simulink model "Proj2_P1"  (Simulink 8.6)
settings: Solver=ode45  StartTime=0.0  StopTime=25  MaxStep=0.001  RelTol=1e-3
values from neighbouring files (symbols this model uses):
  fl_rd_0 = fl_rd_rated    [Proj2_IM_IC_rated.m]    (also in Proj2_P1_calc.m = eps)
  fl_sd_0 = fl_sd_rated    [Proj2_IM_IC_rated.m]    (also in Proj2_P1_calc.m = 0)
  fl_sq_0 = fl_sq_rated    [Proj2_IM_IC_rated.m]    (also in Proj2_P1_calc.m = 0)
  Ia_0 = 0    [Proj2_P1_calc.m]
  IA_0 = 0    [Proj2_P1_calc.m]
  Ib_0 = 0    [Proj2_P1_calc.m]
  IB_0 = 0    [Proj2_P1_calc.m]
  Ic_0 = 0    [Proj2_P1_calc.m]
  IC_0 = 0    [Proj2_P1_calc.m]
  J_eq = 75    [Proj2_IM_parameters.m]
  L_lr = X_lr/w_syn    (= 8.22300539308e-05)    [Proj2_IM_parameters.m]
  L_ls = X_ls/w_syn    (= 9.01878010854e-05)    [Proj2_IM_parameters.m]
  L_m = X_m /w_syn    (= 0.00152788745368)    [Proj2_IM_parameters.m]
  L_r = L_lr+L_m    (= 0.00161011750761)    [Proj2_IM_parameters.m]
  L_s = L_ls+L_m    (= 0.00161807525477)    [Proj2_IM_parameters.m]
  p = 6    [Proj2_IM_parameters.m]
  R_r = 0.991*10^-3    (= 0.000991)    [Proj2_IM_parameters.m]
  R_s = 1.4*10^-3    (= 0.0014)    [Proj2_IM_parameters.m]
  T_L_0 = T_L_rated    [Proj2_IM_IC_rated.m]    (also in Proj2_P1_calc.m = 0)
  T_L_rated = T_em_rated    [Proj2_IM_parameters.m]
  tau_r = L_r/R_r    (= 1.62474016914)    [Proj2_IM_parameters.m]
  theta_Aa_0 = 0    [Proj2_P1_calc.m]
  theta_da_0 = theta_fl_rated_a    [Proj2_IM_IC_rated.m]    (also in Proj2_P1_calc.m = 0)
  theta_dA_0 = theta_fl_rated_a    [Proj2_IM_IC_rated.m]    (also in Proj2_P1_calc.m = 0)
  V_ll_rated = 575    [Proj2_IM_parameters.m]
  Va_0 = 0    [Proj2_P1_calc.m]
  Vb_0 = 0    [Proj2_P1_calc.m]
  Vc_0 = 0    [Proj2_P1_calc.m]
  w_mech_0 = w_mech_rated    [Proj2_IM_IC_rated.m]    (also in Proj2_P1_calc.m = 0)
libraries: aerolibutil x8
settings Model: Creator=XP  LastModifiedBy=XP
settings DataIOCC: SaveFormat=Dataset  SignalLoggingSaveFormat=Dataset
settings OptimizationCC: ExpressionDepthLimit=128
settings DebuggingCC: UnderspecifiedInitializationDetection=Simplified  MergeDetectMultiDrivingBlocksExec=error  SolverPrmCheckMsg=none  FcnCallInpInsideContextMsg=EnableAllAsError  StateNameClashWarn=none
settings HardwareCC: ProdBitPerPointer=64  ProdLargestAtomicFloat=Float  ProdIntDivRoundTo=Zero  ProdEndianess=LittleEndian  ProdWordSize=64  ProdHWDeviceType=Intel->x86-64 (Windows64)
settings GRTTargetCC: GeneratePreprocessorConditionals=Use local settings  CombineOutputUpdateFcns=on  GRTInterface=off
settings ConfigComp: CovModelRefEnable=off

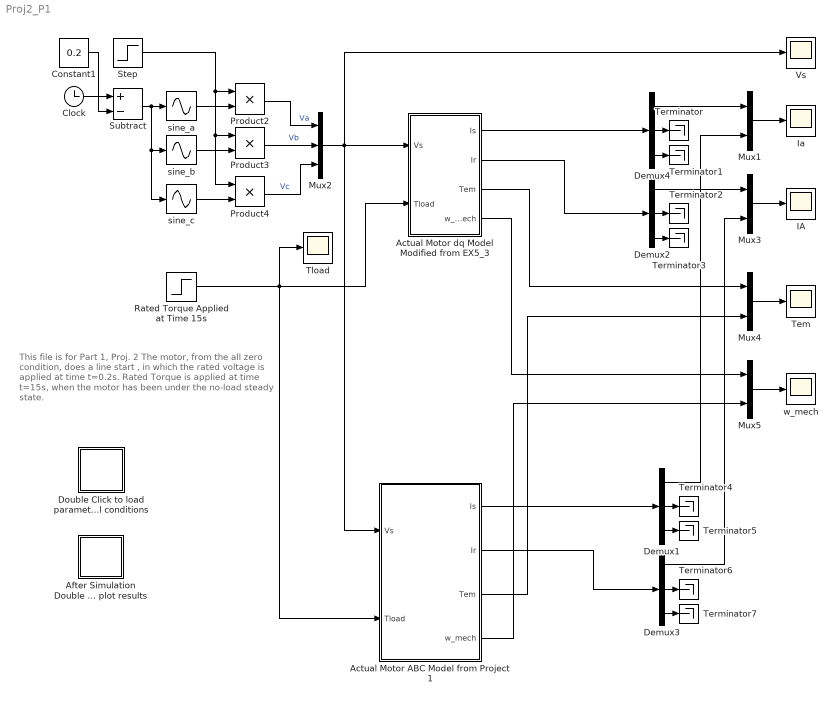
== system Proj2_P1 ==
  note: This file is for Part 1, Proj. 2
      |
      | The motor, from the all zero condition, does a line start ,
      | in which the rated voltage is applied at time t=0.2s.
      |
      | Rated Torque is applied at time t=15s,
      | when the motor has been under the no-load steady state.
  "Actual Motor ABC Model from Project 1 " : Subsystem
  Actual Motor dq Model Modified from EX5_3 : Subsystem
  After Simulation Double Click to plot results : Subsystem
      settings: OpenFcn=Proj2_P1_plots
      mask Display:
      | plot(0,0)
      | plot(100,100)
      | disp('Plot')
  Clock : Clock
  Constant1 : Constant  Value=0.2
  Demux{1..4} (4 alike) : Demux  Outputs=3
  Double Click to load parameters and initial conditions : Subsystem
      settings: OpenFcn=Proj2_P1_calc
      mask Display:
      | plot(0,0)
      | plot(100,100)
      | disp('Start')
  IA : Scope
  Ia : Scope
  Mux{1,3..5} (4 alike) : Mux  Inputs=2
  Mux2 : Mux  Inputs=3
  Product2 : Product
  Product3 : Product
  Product4 : Product
  Rated Torque Applied at Time 15s : Step  Time=15  Before=T_L_0  After=T_L_rated  SampleTime=0
  Step : Step  Time=0.2  SampleTime=0
  Subtract : Sum  Inputs=+-
  Tem : Scope
  Terminator{,1..7} (8 alike) : Terminator
  Tload : Scope
  Vs : Scope
  sine_a : Sin  TimeSource=Use external signal  Amplitude=V_ll_rated*sqrt(2/3)  Frequency=60*2*pi  Phase=pi/2  SampleTime=0
  sine_b : Sin  TimeSource=Use external signal  Amplitude=V_ll_rated*sqrt(2/3)  Frequency=60*2*pi  Phase=pi/2-2*pi/3  SampleTime=0
  sine_c : Sin  TimeSource=Use external signal  Amplitude=V_ll_rated*sqrt(2/3)  Frequency=60*2*pi  Phase=pi/2-4*pi/3  SampleTime=0
  w_mech : Scope
  wires:
  Subtract/1 -> sine_c/1, sine_b/1, sine_a/1
  Step/1 -> Product3/1, Product4/1, Product2/1
  sine_a/1 -> Product2/2
  Product2/1 -> Mux2/1  "Va"
  sine_c/1 -> Product4/2
  sine_b/1 -> Product3/2
  Product3/1 -> Mux2/2  "Vb"
  Product4/1 -> Mux2/3  "Vc"
  Clock/1 -> Subtract/1
  Constant1/1 -> Subtract/2
  Mux2/1 -> "Actual Motor ABC Model from Project 1 "/1(Vs), Actual Motor dq Model Modified from EX5_3/1(Vs), Vs/1
  Rated Torque Applied at Time 15s/1 -> Tload/1, Actual Motor dq Model Modified from EX5_3/2(Tload), "Actual Motor ABC Model from Project 1 "/2(Tload)
  Actual Motor dq Model Modified from EX5_3/1(Is) -> Demux4/1
  "Actual Motor ABC Model from Project 1 "/1(Is) -> Demux1/1
  Actual Motor dq Model Modified from EX5_3/2(Ir) -> Demux2/1
  "Actual Motor ABC Model from Project 1 "/2(Ir) -> Demux3/1
  Demux4/1 -> Mux1/1
  Demux1/1 -> Mux1/2
  Mux1/1 -> Ia/1
  Actual Motor dq Model Modified from EX5_3/3(Tem) -> Mux4/1
  "Actual Motor ABC Model from Project 1 "/3(Tem) -> Mux4/2
  Mux4/1 -> Tem/1
  Mux5/1 -> w_mech/1
  Actual Motor dq Model Modified from EX5_3/4(w_mech) -> Mux5/1
  "Actual Motor ABC Model from Project 1 "/4(w_mech) -> Mux5/2
  Mux3/1 -> IA/1
  Demux2/1 -> Mux3/1
  Demux3/1 -> Mux3/2
  Demux4/2 -> Terminator/1
  Demux4/3 -> Terminator1/1
  Demux2/2 -> Terminator2/1
  Demux2/3 -> Terminator3/1
  Demux1/2 -> Terminator4/1
  Demux1/3 -> Terminator5/1
  Demux3/2 -> Terminator6/1
  Demux3/3 -> Terminator7/1

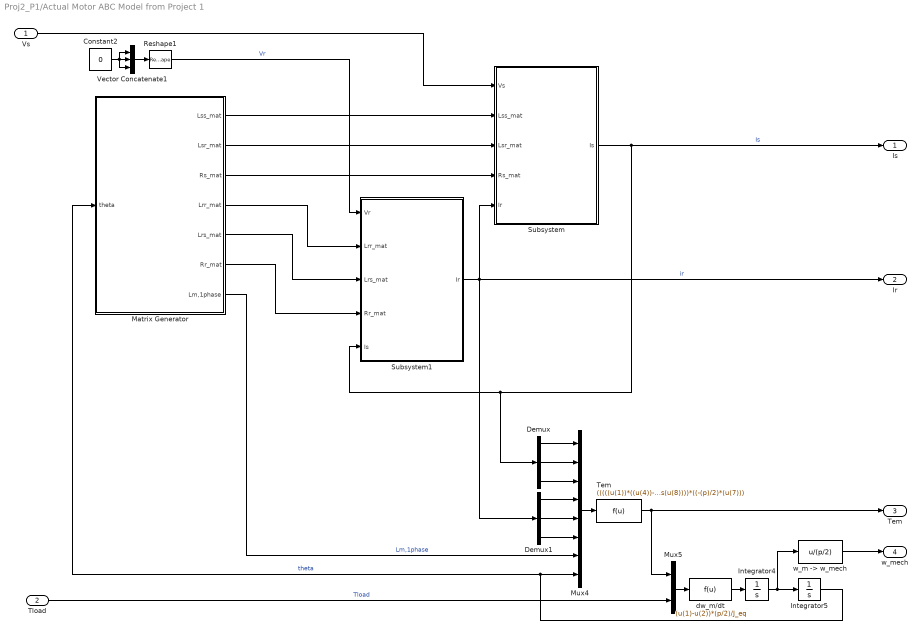
== system Proj2_P1/Actual Motor ABC Model from Project 1  ==
  Vs : Inport
  Tload : Inport  Port=2
  Constant2 : Constant  Value=0
  Demux : Demux  Outputs=3
  Demux1 : Demux  Outputs=3
  Integrator4 : Integrator  InitialCondition=w_mech_0*p/2
  Integrator5 : Integrator  InitialCondition=theta_Aa_0
  Matrix Generator : Subsystem
  Mux4 : Mux  Inputs=8
  Mux5 : Mux  Inputs=2
  Reshape1 : Reshape  OutputDimensionality=Customize  OutputDimensions=[3,1]
  Subsystem : Subsystem
  Subsystem1 : Subsystem
  "Tem " : Fcn  Expr=(((((u(1))*((u(4))-(0.5*(u(5)))-(0.5*(u(6)))))+((u(2))*((u(5))-(0.5*(u(4)))-(0.5*(u(6)))))+((u(3))*((u(6))-(0.5*(u(5)))-(0.5*(u(4))))))*sin(u(8)))+((sqrt(3)/2)*(((u(1))*((u(5))-(u(6))))+((u(2))*((u(6))-(u(4))))+((u(3))*((u(4))-(u(5)))))*cos(u(8))))*((-(p)/2)*(u(7)))
  Vector Concatenate1 : Concatenate  NumInputs=3
  dw_m/dt : Fcn  Expr=(u(1)-u(2))*(p/2)/J_eq
  "w_m -> w_mech" : Fcn  Expr=u/(p/2)
  Is : Outport
  Ir : Outport  Port=2
  Tem : Outport  Port=3
  w_mech : Outport  Port=4
  wires:
  Matrix Generator/7(Lm,1phase) -> Mux4/7  "Lm,1phase"
  Tload/1 -> Mux5/2  "Tload"
  Subsystem1/1(Ir) -> Ir/1, Demux1/1, Subsystem/5(Ir)  "ir"
  Integrator5/1 -> Mux4/8, Matrix Generator/1(theta)  "theta"
  Vector Concatenate1/1 -> Reshape1/1
  Reshape1/1 -> Subsystem1/1(Vr)  "Vr"
  Matrix Generator/5(Lrs_mat) -> Subsystem1/3(Lrs_mat)
  "w_m -> w_mech"/1 -> w_mech/1
  Demux/3 -> Mux4/3
  Demux1/1 -> Mux4/4
  Mux5/1 -> dw_m/dt/1
  Constant2/1 -> Vector Concatenate1/3, Vector Concatenate1/1, Vector Concatenate1/2
  Subsystem/1(Is) -> Is/1, Demux/1, Subsystem1/5(Is)  "Is"
  Matrix Generator/6(Rr_mat) -> Subsystem1/4(Rr_mat)
  Matrix Generator/4(Lrr_mat) -> Subsystem1/2(Lrr_mat)
  Demux1/2 -> Mux4/5
  Demux1/3 -> Mux4/6
  Mux4/1 -> "Tem "/1
  "Tem "/1 -> Tem/1, Mux5/1
  Demux/1 -> Mux4/1
  Demux/2 -> Mux4/2
  Integrator4/1 -> "w_m -> w_mech"/1, Integrator5/1
  dw_m/dt/1 -> Integrator4/1
  Matrix Generator/1(Lss_mat) -> Subsystem/2(Lss_mat)
  Matrix Generator/3(Rs_mat) -> Subsystem/4(Rs_mat)
  Matrix Generator/2(Lsr_mat) -> Subsystem/3(Lsr_mat)
  Vs/1 -> Subsystem/1(Vs)

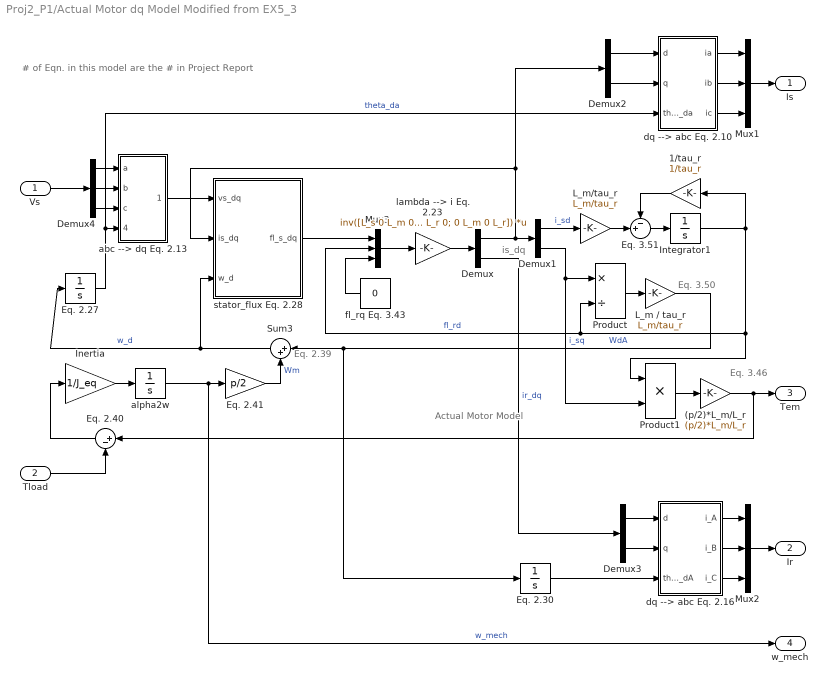
== system Proj2_P1/Actual Motor dq Model Modified from EX5_3 ==
  note: Eq. 2.39
  note: Eq. 3.46
  note: Eq. 3.50
  note: # of Eqn. in this model are the # in Project Report
  note: Actual Motor Model
  note: is_dq
  Vs : Inport
  Tload : Inport  Port=2
  (p/2)*L_m/L_r : Gain  Gain=(p/2)*L_m/L_r  SaturateOnIntegerOverflow=on  OutDataTypeStr=Inherit: Same as input  ParamDataTypeStr=Inherit: Same as input
  1/tau_r : Gain  Gain=1/tau_r  SaturateOnIntegerOverflow=on  OutDataTypeStr=Inherit: Same as input  ParamDataTypeStr=Inherit: Same as input
  Demux{,1..3} (4 alike) : Demux  Outputs=2
  Demux4 : Demux  Outputs=3
  Eq. 2.27 : Integrator  InitialCondition=theta_da_0
  Eq. 2.30 : Integrator  InitialCondition=theta_dA_0
  Eq. 2.40 : Sum  Inputs=|+-  SaturateOnIntegerOverflow=on  InputSameDT=on  OutDataTypeStr=Inherit: Same as first input
  Eq. 2.41 : Gain  Gain=p/2  SaturateOnIntegerOverflow=on  OutDataTypeStr=Inherit: Same as input  ParamDataTypeStr=Inherit: Same as input
  Eq. 3.51 : Sum  Inputs=-+|  SaturateOnIntegerOverflow=on  InputSameDT=on  OutDataTypeStr=Inherit: Same as first input
  Inertia : Gain  Gain=1/J_eq  SaturateOnIntegerOverflow=on  OutDataTypeStr=Inherit: Same as input  ParamDataTypeStr=Inherit: Same as input
  Integrator1 : Integrator  InitialCondition=fl_rd_0
  L_m / tau_r : Gain  Gain=L_m/tau_r  SaturateOnIntegerOverflow=on  OutDataTypeStr=Inherit: Same as input  ParamDataTypeStr=Inherit: Same as input
  L_m/tau_r : Gain  Gain=L_m/tau_r  SaturateOnIntegerOverflow=on  OutDataTypeStr=Inherit: Same as input  ParamDataTypeStr=Inherit: Same as input
  Mux1 : Mux  Inputs=3
  Mux2 : Mux  Inputs=3
  Mux3 : Mux  Inputs=3
  Product : Product  Inputs=*/  SaturateOnIntegerOverflow=on  RndMeth=Zero  InputSameDT=on  OutDataTypeStr=Inherit: Same as first input
  Product1 : Product  SaturateOnIntegerOverflow=on  RndMeth=Zero  InputSameDT=on  OutDataTypeStr=Inherit: Same as first input
  Sum3 : Sum  Inputs=|++  SaturateOnIntegerOverflow=on  InputSameDT=on  OutDataTypeStr=Inherit: Same as first input
  abc --> dq Eq. 2.13 : Subsystem
  alpha2w : Integrator  InitialCondition=w_mech_0
  dq --> abc Eq. 2.10 : Subsystem
  "dq --> abc Eq. 2.16 " : Subsystem
  fl_rq Eq. 3.43 : Constant  Value=0
  lambda --> i Eq. 2.23 : Gain  Gain=inv([L_s 0 L_m 0; 0 L_s 0 L_m; L_m 0 L_r 0; 0 L_m 0 L_r])  Multiplication=Matrix(K*u)  SaturateOnIntegerOverflow=on  OutDataTypeStr=Inherit: Same as input  ParamDataTypeStr=Inherit: Same as input
  stator_flux Eq. 2.28 : Subsystem
  Is : Outport
  Ir : Outport  Port=2
  Tem : Outport  Port=3
  w_mech : Outport  Port=4
  wires:
  Mux3/1 -> lambda --> i Eq. 2.23/1
  Demux/1 -> Demux1/1, stator_flux Eq. 2.28/2(is_dq), Demux2/1
  Eq. 2.27/1 -> dq --> abc Eq. 2.10/3(theta_da), abc --> dq Eq. 2.13/4(theta_da)  "theta_da"
  stator_flux Eq. 2.28/1(fl_s_dq) -> Mux3/1
  abc --> dq Eq. 2.13/1(vs_dq) -> stator_flux Eq. 2.28/1(vs_dq)
  lambda --> i Eq. 2.23/1 -> Demux/1
  Demux1/1 -> L_m/tau_r/1  "i_sd"
  L_m/tau_r/1 -> Eq. 3.51/2
  1/tau_r/1 -> Eq. 3.51/1
  Eq. 3.51/1 -> Integrator1/1
  Demux1/2 -> Product/1, Product1/2  "i_sq"
  Product/1 -> L_m / tau_r/1
  L_m / tau_r/1 -> Sum3/1, Eq. 2.30/1  "WdA"
  Product1/1 -> (p/2)*L_m/L_r/1
  fl_rq Eq. 3.43/1 -> Mux3/3
  Sum3/1 -> Eq. 2.27/1, stator_flux Eq. 2.28/3(w_d)  "w_d"
  (p/2)*L_m/L_r/1 -> Tem/1, Eq. 2.40/1
  Demux2/1 -> dq --> abc Eq. 2.10/1(d)
  Demux2/2 -> dq --> abc Eq. 2.10/2(q)
  dq --> abc Eq. 2.10/1(ia) -> Mux1/1
  dq --> abc Eq. 2.10/2(ib) -> Mux1/2
  dq --> abc Eq. 2.10/3(ic) -> Mux1/3
  Integrator1/1 -> 1/tau_r/1, Mux3/2, Product/2, Product1/1  "fl_rd"
  Eq. 2.41/1 -> Sum3/2  "Wm"
  Demux/2 -> Demux3/1  "ir_dq"
  Eq. 2.40/1 -> Inertia/1
  Inertia/1 -> alpha2w/1
  alpha2w/1 -> w_mech/1, Eq. 2.41/1  "w_mech"
  Tload/1 -> Eq. 2.40/2
  Mux1/1 -> Is/1
  Demux3/1 -> "dq --> abc Eq. 2.16 "/1(d)
  Demux3/2 -> "dq --> abc Eq. 2.16 "/2(q)
  Eq. 2.30/1 -> "dq --> abc Eq. 2.16 "/3(theta_dA)
  "dq --> abc Eq. 2.16 "/1(i_A) -> Mux2/1
  "dq --> abc Eq. 2.16 "/2(i_B) -> Mux2/2
  "dq --> abc Eq. 2.16 "/3(i_C) -> Mux2/3
  Mux2/1 -> Ir/1
  Demux4/1 -> abc --> dq Eq. 2.13/1(a)
  Demux4/2 -> abc --> dq Eq. 2.13/2(b)
  Demux4/3 -> abc --> dq Eq. 2.13/3(c)
  Vs/1 -> Demux4/1

== system Proj2_P1/After Simulation Double Click to plot results ==

== system Proj2_P1/Double Click to load parameters and initial conditions ==

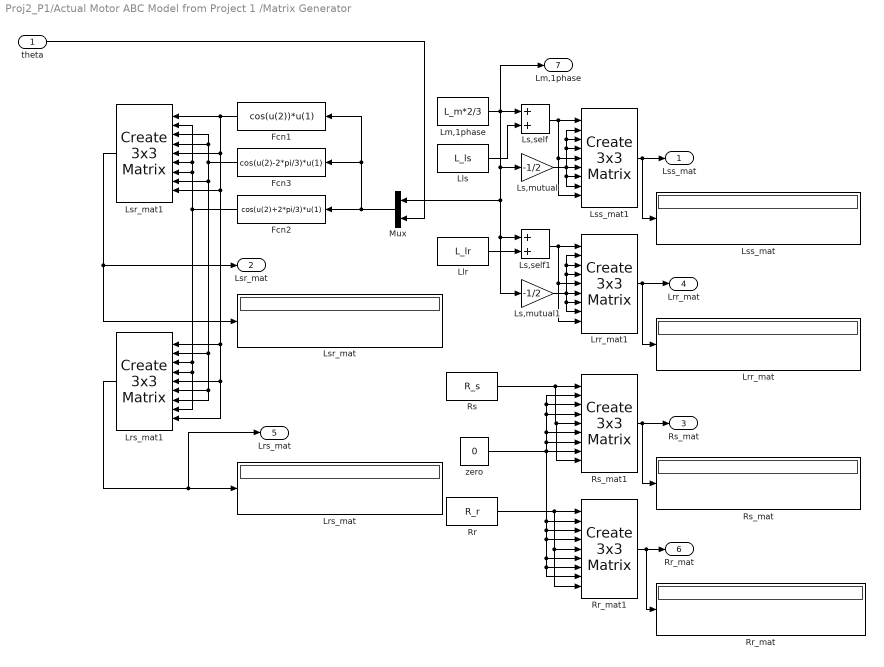
== system Proj2_P1/Actual Motor ABC Model from Project 1 /Matrix Generator ==
  theta : Inport
  Fcn1 : Fcn  Expr=cos(u(2))*u(1)
  Fcn2 : Fcn  Expr=cos(u(2)+2*pi/3)*u(1)
  Fcn3 : Fcn  Expr=cos(u(2)-2*pi/3)*u(1)
  Llr : Constant  Value=L_lr
  Lls : Constant  Value=L_ls
  "Lm,1phase " : Constant  Value=L_m*2/3
  "Lrr_mat " : Display
  Lrr_mat1 : aerolibutil/Create 3x3 Matrix
  "Lrs_mat " : Display
  Lrs_mat1 : aerolibutil/Create 3x3 Matrix
  Ls,mutual : Gain  Gain=-1/2
  Ls,mutual1 : Gain  Gain=-1/2
  Ls,self : Sum
  Ls,self1 : Sum
  "Lsr_mat " : Display
  Lsr_mat1 : aerolibutil/Create 3x3 Matrix
  "Lss_mat " : Display
  Lss_mat1 : aerolibutil/Create 3x3 Matrix
  Mux : Mux  Inputs=2
  "Rr " : Constant  Value=R_r
  "Rr_mat " : Display
  Rr_mat1 : aerolibutil/Create 3x3 Matrix
  Rs : Constant  Value=R_s
  "Rs_mat " : Display
  Rs_mat1 : aerolibutil/Create 3x3 Matrix
  "zero " : Constant  Value=0
  Lss_mat : Outport
  Lsr_mat : Outport  Port=2
  Rs_mat : Outport  Port=3
  Lrr_mat : Outport  Port=4
  Lrs_mat : Outport  Port=5
  Rr_mat : Outport  Port=6
  Lm,1phase : Outport  Port=7
  wires:
  Ls,self/1 -> Lss_mat1/1, Lss_mat1/9, Lss_mat1/5
  Lls/1 -> Ls,self/2
  Lsr_mat1/1 -> Lsr_mat/1, "Lsr_mat "/1
  Mux/1 -> Fcn3/1, Fcn1/1, Fcn2/1
  Rs/1 -> Rs_mat1/9, Rs_mat1/5, Rs_mat1/1
  "Rr "/1 -> Rr_mat1/9, Rr_mat1/5, Rr_mat1/1
  Lrs_mat1/1 -> Lrs_mat/1, "Lrs_mat "/1
  Fcn1/1 -> Lrs_mat1/1, Lrs_mat1/5, Lrs_mat1/9, Lsr_mat1/9, Lsr_mat1/5, Lsr_mat1/1
  Lrr_mat1/1 -> Lrr_mat/1, "Lrr_mat "/1
  Ls,mutual/1 -> Lss_mat1/8, Lss_mat1/7, Lss_mat1/4, Lss_mat1/3, Lss_mat1/2, Lss_mat1/6
  Rr_mat1/1 -> Rr_mat/1, "Rr_mat "/1
  Ls,self1/1 -> Lrr_mat1/9, Lrr_mat1/5, Lrr_mat1/1
  "zero "/1 -> Rs_mat1/4, Rs_mat1/3, Rs_mat1/2, Rs_mat1/6, Rs_mat1/7, Rr_mat1/2, Rr_mat1/3, Rr_mat1/4, Rr_mat1/6, Rr_mat1/7, Rr_mat1/8, Rs_mat1/8
  Fcn3/1 -> Lrs_mat1/7, Lrs_mat1/6, Lrs_mat1/2, Lsr_mat1/8, Lsr_mat1/4, Lsr_mat1/3
  Llr/1 -> Ls,self1/2
  Rs_mat1/1 -> Rs_mat/1, "Rs_mat "/1
  Ls,mutual1/1 -> Lrr_mat1/8, Lrr_mat1/7, Lrr_mat1/4, Lrr_mat1/3, Lrr_mat1/2, Lrr_mat1/6
  Fcn2/1 -> Lsr_mat1/7, Lsr_mat1/6, Lsr_mat1/2, Lrs_mat1/8, Lrs_mat1/4, Lrs_mat1/3
  theta/1 -> Mux/2
  "Lm,1phase "/1 -> Lm,1phase/1, Mux/1, Ls,self1/1, Ls,mutual1/1, Ls,mutual/1, Ls,self/1
  Lss_mat1/1 -> Lss_mat/1, "Lss_mat "/1

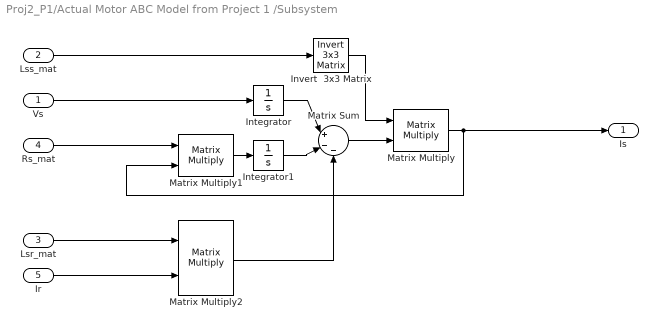
== system Proj2_P1/Actual Motor ABC Model from Project 1 /Subsystem ==
  Vs : Inport
  Lss_mat : Inport  Port=2
  Lsr_mat : Inport  Port=3
  Rs_mat : Inport  Port=4
  Ir : Inport  Port=5
  Integrator : Integrator  InitialCondition=[Va_0;Vb_0;Vc_0]
  Integrator1 : Integrator  InitialCondition=R_s*eye(3)*[Ia_0;Ib_0;Ic_0]
  Invert  3x3 Matrix : aerolibutil/Invert  3x3 Matrix
  Matrix Sum : Sum  Inputs=|+--
  Matrix Multiply : Product  Multiplication=Matrix(*)
  Matrix Multiply1 : Product  Multiplication=Matrix(*)
  Matrix Multiply2 : Product  Multiplication=Matrix(*)
  Is : Outport
  wires:
  Matrix Sum/1 -> Matrix Multiply/2
  Matrix Multiply/1 -> Is/1, Matrix Multiply1/2
  Matrix Multiply2/1 -> Matrix Sum/3
  Lss_mat/1 -> Invert  3x3 Matrix/1
  Vs/1 -> Integrator/1
  Invert  3x3 Matrix/1 -> Matrix Multiply/1
  Integrator/1 -> Matrix Sum/1
  Lsr_mat/1 -> Matrix Multiply2/1
  Matrix Multiply1/1 -> Integrator1/1
  Integrator1/1 -> Matrix Sum/2
  Rs_mat/1 -> Matrix Multiply1/1
  Ir/1 -> Matrix Multiply2/2

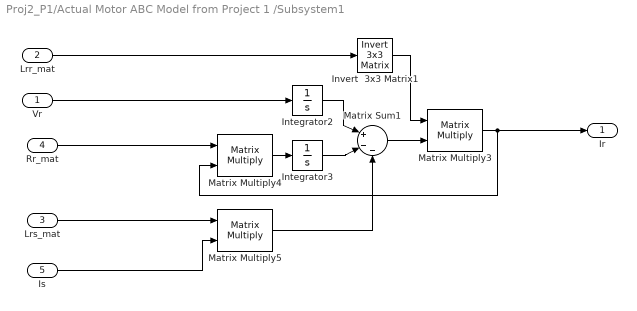
== system Proj2_P1/Actual Motor ABC Model from Project 1 /Subsystem1 ==
  Vr : Inport
  Lrr_mat : Inport  Port=2
  Lrs_mat : Inport  Port=3
  Rr_mat : Inport  Port=4
  Is : Inport  Port=5
  Integrator2 : Integrator
  Integrator3 : Integrator  InitialCondition=R_r*eye(3)*[IA_0;IB_0;IC_0]
  Invert  3x3 Matrix1 : aerolibutil/Invert  3x3 Matrix
  Matrix Sum1 : Sum  Inputs=|+--
  Matrix Multiply3 : Product  Multiplication=Matrix(*)
  Matrix Multiply4 : Product  Multiplication=Matrix(*)
  Matrix Multiply5 : Product  Multiplication=Matrix(*)
  Ir : Outport
  wires:
  Integrator3/1 -> Matrix Sum1/2
  Rr_mat/1 -> Matrix Multiply4/1
  Matrix Multiply4/1 -> Integrator3/1
  Is/1 -> Matrix Multiply5/2
  Invert  3x3 Matrix1/1 -> Matrix Multiply3/1
  Matrix Sum1/1 -> Matrix Multiply3/2
  Matrix Multiply3/1 -> Ir/1, Matrix Multiply4/2
  Integrator2/1 -> Matrix Sum1/1
  Vr/1 -> Integrator2/1
  Lrr_mat/1 -> Invert  3x3 Matrix1/1
  Lrs_mat/1 -> Matrix Multiply5/1
  Matrix Multiply5/1 -> Matrix Sum1/3

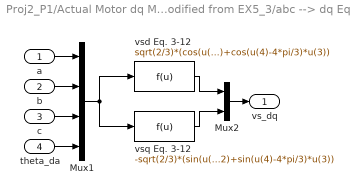
== system Proj2_P1/Actual Motor dq Model Modified from EX5_3/abc --> dq Eq. 2.13 ==
  a : Inport
  b : Inport  Port=2
  c : Inport  Port=3
  theta_da : Inport  Port=4
  Mux1 : Mux
  Mux2 : Mux  Inputs=2
  vsd Eq. 3-12 : Fcn  Expr=sqrt(2/3)*(cos(u(4))*u(1)+cos(u(4)-2*pi/3)*u(2)+cos(u(4)-4*pi/3)*u(3))
  vsq Eq. 3-12 : Fcn  Expr=-sqrt(2/3)*(sin(u(4))*u(1)+sin(u(4)-2*pi/3)*u(2)+sin(u(4)-4*pi/3)*u(3))
  vs_dq : Outport
  wires:
  Mux1/1 -> vsd Eq. 3-12/1, vsq Eq. 3-12/1
  vsd Eq. 3-12/1 -> Mux2/1
  vsq Eq. 3-12/1 -> Mux2/2
  a/1 -> Mux1/1
  b/1 -> Mux1/2
  c/1 -> Mux1/3
  theta_da/1 -> Mux1/4
  Mux2/1 -> vs_dq/1

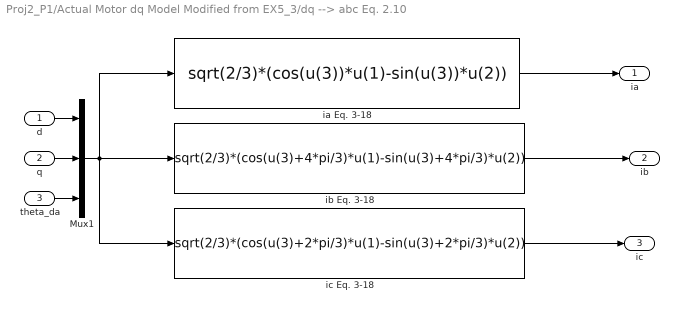
== system Proj2_P1/Actual Motor dq Model Modified from EX5_3/dq --> abc Eq. 2.10 ==
  d : Inport
  q : Inport  Port=2
  theta_da : Inport  Port=3
  Mux1 : Mux  Inputs=3
  ia Eq. 3-18 : Fcn  Expr=sqrt(2/3)*(cos(u(3))*u(1)-sin(u(3))*u(2))
  ib Eq. 3-18 : Fcn  Expr=sqrt(2/3)*(cos(u(3)+4*pi/3)*u(1)-sin(u(3)+4*pi/3)*u(2))
  ic Eq. 3-18 : Fcn  Expr=sqrt(2/3)*(cos(u(3)+2*pi/3)*u(1)-sin(u(3)+2*pi/3)*u(2))
  ia : Outport
  ib : Outport  Port=2
  ic : Outport  Port=3
  wires:
  ic Eq. 3-18/1 -> ic/1
  Mux1/1 -> ic Eq. 3-18/1, ib Eq. 3-18/1, ia Eq. 3-18/1
  ia Eq. 3-18/1 -> ia/1
  ib Eq. 3-18/1 -> ib/1
  d/1 -> Mux1/1
  q/1 -> Mux1/2
  theta_da/1 -> Mux1/3

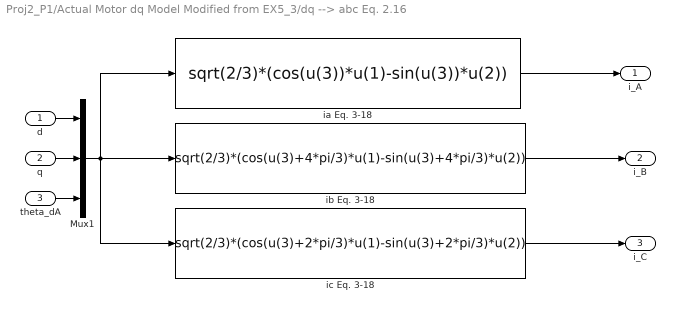
== system Proj2_P1/Actual Motor dq Model Modified from EX5_3/dq --> abc Eq. 2.16  ==
  d : Inport
  q : Inport  Port=2
  theta_dA : Inport  Port=3
  Mux1 : Mux  Inputs=3
  ia Eq. 3-18 : Fcn  Expr=sqrt(2/3)*(cos(u(3))*u(1)-sin(u(3))*u(2))
  ib Eq. 3-18 : Fcn  Expr=sqrt(2/3)*(cos(u(3)+4*pi/3)*u(1)-sin(u(3)+4*pi/3)*u(2))
  ic Eq. 3-18 : Fcn  Expr=sqrt(2/3)*(cos(u(3)+2*pi/3)*u(1)-sin(u(3)+2*pi/3)*u(2))
  i_A : Outport
  i_B : Outport  Port=2
  i_C : Outport  Port=3
  wires:
  ic Eq. 3-18/1 -> i_C/1
  Mux1/1 -> ic Eq. 3-18/1, ib Eq. 3-18/1, ia Eq. 3-18/1
  ib Eq. 3-18/1 -> i_B/1
  d/1 -> Mux1/1
  q/1 -> Mux1/2
  theta_dA/1 -> Mux1/3
  ia Eq. 3-18/1 -> i_A/1

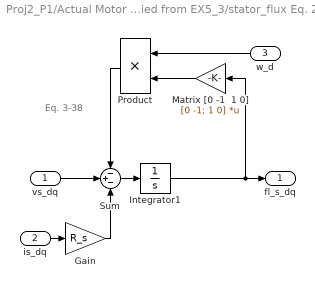
== system Proj2_P1/Actual Motor dq Model Modified from EX5_3/stator_flux Eq. 2.28 ==
  note: Eq. 3-38
  vs_dq : Inport
  is_dq : Inport  Port=2
  w_d : Inport  Port=3
  Gain : Gain  Gain=R_s  SaturateOnIntegerOverflow=on  OutDataTypeStr=Inherit: Same as input  ParamDataTypeStr=Inherit: Same as input
  Integrator1 : Integrator  InitialCondition=[fl_sd_0; fl_sq_0]
  "Matrix [0 -1  1 0] " : Gain  Gain=[0 -1; 1 0]  Multiplication=Matrix(K*u)  SaturateOnIntegerOverflow=on  OutDataTypeStr=Inherit: Same as input  ParamDataTypeStr=Inherit: Same as input
  Product : Product  SaturateOnIntegerOverflow=on  RndMeth=Zero  InputSameDT=on  OutDataTypeStr=Inherit: Same as first input
  Sum : Sum  Inputs=-+-  SaturateOnIntegerOverflow=on  InputSameDT=on  OutDataTypeStr=Inherit: Same as first input
  fl_s_dq : Outport
  wires:
  Sum/1 -> Integrator1/1
  Integrator1/1 -> "Matrix [0 -1  1 0] "/1, fl_s_dq/1
  "Matrix [0 -1  1 0] "/1 -> Product/2
  Product/1 -> Sum/1
  w_d/1 -> Product/1
  vs_dq/1 -> Sum/2
  is_dq/1 -> Gain/1
  Gain/1 -> Sum/3
